simulink library "roller485lib"  (R2023a)
settings: Solver=VariableStepAuto  StartTime=0.0  StopTime=10.0  RelTol=1e-3
libraries: arduinolib x135, simulink x46
(part 4 of 4)

== matlab function roller485lib/I2C Write (using MATLAB Function)/current command [mA] (using MATLAB Function)/MATLAB Function ==
  data: double_data input; bytes output
function bytes = double_to_bytes_uint8(double_data)

bytes        = zeros(1, 4, 'uint8');             % 明示的に型とサイズを宣言
signed_int   = int32(double_data);
unsigned_int = typecast(signed_int, 'uint32');
bytes(1:4)   = typecast(unsigned_int, 'uint8');  % サイズを明示

== matlab function roller485lib/I2C Write (using MATLAB Function)/relative angle command [deg] (using MATLAB Function)/Enabled Subsystem (initialization angle)/MATLAB Function ==
  data: bytes input; double_data output
function double_data = bytes_uint8_to_double(bytes)

double_data    = zeros(1, 1, 'double');    % 明示的に型とサイズを宣言
unsigned_int   = typecast(uint8(bytes), 'uint32');
signed_int     = typecast(unsigned_int, 'int32');
double_data(1) = double(signed_int);       % サイズを明示

== matlab function roller485lib/I2C Write/relative angle command [rad]/Enabled Subsystem (initialization angle)/MATLAB Function ==
  data: bytes input; double_data output
function double_data = bytes_uint8_to_double(bytes)

double_data    = zeros(1, 1, 'double');    % 明示的に型とサイズを宣言
unsigned_int   = typecast(uint8(bytes), 'uint32');
signed_int     = typecast(unsigned_int, 'int32');
double_data(1) = double(signed_int);       % サイズを明示

== matlab function roller485lib/I2C Write (using MATLAB Function)/relative angle command [deg] (using MATLAB Function)/MATLAB Function ==
  data: double_data input; bytes output
function bytes = double_to_bytes_uint8(double_data)

bytes        = zeros(1, 4, 'uint8');             % 明示的に型とサイズを宣言
signed_int   = int32(double_data);
unsigned_int = typecast(signed_int, 'uint32');
bytes(1:4)   = typecast(unsigned_int, 'uint8');  % サイズを明示

== matlab function roller485lib/I2C Write (using MATLAB Function)/relative angle command [rad] (using MATLAB Function)/Enabled Subsystem (initialization angle)/MATLAB Function ==
  data: bytes input; double_data output
function double_data = bytes_uint8_to_double(bytes)

double_data    = zeros(1, 1, 'double');    % 明示的に型とサイズを宣言
unsigned_int   = typecast(uint8(bytes), 'uint32');
signed_int     = typecast(unsigned_int, 'int32');
double_data(1) = double(signed_int);       % サイズを明示

== matlab function roller485lib/I2C Write (using MATLAB Function)/relative angle command [rad] (using MATLAB Function)/MATLAB Function ==
  data: double_data input; bytes output
function bytes = double_to_bytes_uint8(double_data)

bytes        = zeros(1, 4, 'uint8');             % 明示的に型とサイズを宣言
signed_int   = int32(double_data);
unsigned_int = typecast(signed_int, 'uint32');
bytes(1:4)   = typecast(unsigned_int, 'uint8');  % サイズを明示

== matlab function roller485lib/I2C Read (using MATLAB Function)/absolute angle detection [rad] (using MATLAB Function)/MATLAB Function ==
  data: bytes input; double_data output
function double_data = bytes_uint8_to_double(bytes)

double_data    = zeros(1, 1, 'double');    % 明示的に型とサイズを宣言
unsigned_int   = typecast(uint8(bytes), 'uint32');
signed_int     = typecast(unsigned_int, 'int32');
double_data(1) = double(signed_int);       % サイズを明示

== matlab function roller485lib/I2C Read (using MATLAB Function)/relative angle detection [rad] (using MATLAB Function)/MATLAB Function ==
  data: bytes input; double_data output
function double_data = bytes_uint8_to_double(bytes)

double_data    = zeros(1, 1, 'double');    % 明示的に型とサイズを宣言
unsigned_int   = typecast(uint8(bytes), 'uint32');
signed_int     = typecast(unsigned_int, 'int32');
double_data(1) = double(signed_int);       % サイズを明示

== matlab function roller485lib/I2C Read (using MATLAB Function)/absolute angle detection [deg] (using MATLAB Function)/MATLAB Function ==
  data: bytes input; double_data output
function double_data = bytes_uint8_to_double(bytes)

double_data    = zeros(1, 1, 'double');    % 明示的に型とサイズを宣言
unsigned_int   = typecast(uint8(bytes), 'uint32');
signed_int     = typecast(unsigned_int, 'int32');
double_data(1) = double(signed_int);       % サイズを明示

== matlab function roller485lib/I2C Write/relative angle command [deg]/Enabled Subsystem (initialization angle)/MATLAB Function ==
  data: bytes input; double_data output
function double_data = bytes_uint8_to_double(bytes)

double_data    = zeros(1, 1, 'double');    % 明示的に型とサイズを宣言
unsigned_int   = typecast(uint8(bytes), 'uint32');
signed_int     = typecast(unsigned_int, 'int32');
double_data(1) = double(signed_int);       % サイズを明示

== matlab function roller485lib/I2C Read (using MATLAB Function)/angular velocity detection using LPF [rpm] (using MATLAB Function)/MATLAB Function2 ==
  data: bytes input; double_data output
function double_data = bytes_uint8_to_double(bytes)

double_data    = zeros(1, 1, 'double');    % 明示的に型とサイズを宣言
unsigned_int   = typecast(uint8(bytes), 'uint32');
signed_int     = typecast(unsigned_int, 'int32');
double_data(1) = double(signed_int);       % サイズを明示

== matlab function roller485lib/I2C Read (using MATLAB Function)/current detection [mA] (using MATLAB Function)/MATLAB Function ==
  data: bytes input; double_data output
function double_data = bytes_uint8_to_double(bytes)

double_data    = zeros(1, 1, 'double');    % 明示的に型とサイズを宣言
unsigned_int   = typecast(uint8(bytes), 'uint32');
signed_int     = typecast(unsigned_int, 'int32');
double_data(1) = double(signed_int);       % サイズを明示

== matlab function roller485lib/I2C Read (using MATLAB Function)/relative angle detection [deg] (using MATLAB Function)/MATLAB Function ==
  data: bytes input; double_data output
function double_data = bytes_uint8_to_double(bytes)

double_data    = zeros(1, 1, 'double');    % 明示的に型とサイズを宣言
unsigned_int   = typecast(uint8(bytes), 'uint32');
signed_int     = typecast(unsigned_int, 'int32');
double_data(1) = double(signed_int);       % サイズを明示

== matlab function roller485lib/Basic I2C Write (using MATLAB Function)/basic relative angle command [rad] (using MATLAB Function)/Enabled Subsystem (initialization angle)/MATLAB Function ==
  data: bytes input; double_data output
function double_data = bytes_uint8_to_double(bytes)

double_data    = zeros(1, 1, 'double');    % 明示的に型とサイズを宣言
unsigned_int   = typecast(uint8(bytes), 'uint32');
signed_int     = typecast(unsigned_int, 'int32');
double_data(1) = double(signed_int);       % サイズを明示

== matlab function roller485lib/Basic I2C Write (using MATLAB Function)/basic relative angle command [rad] (using MATLAB Function)/MATLAB Function ==
  data: double_data input; bytes output
function bytes = double_to_bytes_uint8(double_data)

bytes        = zeros(1, 4, 'uint8');             % 明示的に型とサイズを宣言
signed_int   = int32(double_data);
unsigned_int = typecast(signed_int, 'uint32');
bytes(1:4)   = typecast(unsigned_int, 'uint8');  % サイズを明示

== matlab function roller485lib/Basic I2C Write (using MATLAB Function)/position PID (using MATLAB Function)/MATLAB Function (D) ==
  data: double_data input; bytes output
function bytes = double_to_bytes_uint8(double_data)

bytes        = zeros(1, 4, 'uint8');             % 明示的に型とサイズを宣言
signed_int   = int32(double_data);
unsigned_int = typecast(signed_int, 'uint32');
bytes(1:4)   = typecast(unsigned_int, 'uint8');  % サイズを明示

== matlab function roller485lib/Basic I2C Write (using MATLAB Function)/position PID (using MATLAB Function)/MATLAB Function (I) ==
  data: double_data input; bytes output
function bytes = double_to_bytes_uint8(double_data)

bytes        = zeros(1, 4, 'uint8');             % 明示的に型とサイズを宣言
signed_int   = int32(double_data);
unsigned_int = typecast(signed_int, 'uint32');
bytes(1:4)   = typecast(unsigned_int, 'uint8');  % サイズを明示

== matlab function roller485lib/Basic I2C Write (using MATLAB Function)/position PID (using MATLAB Function)/MATLAB Function (P) ==
  data: double_data input; bytes output
function bytes = double_to_bytes_uint8(double_data)

bytes        = zeros(1, 4, 'uint8');             % 明示的に型とサイズを宣言
signed_int   = int32(double_data);
unsigned_int = typecast(signed_int, 'uint32');
bytes(1:4)   = typecast(unsigned_int, 'uint8');  % サイズを明示

== matlab function roller485lib/Basic I2C Write (using MATLAB Function)/position PID (within set time) (using MATLAB Function)/Enabled Subsystem/MATLAB Function (D) ==
  data: double_data input; bytes output
function bytes = double_to_bytes_uint8(double_data)

bytes        = zeros(1, 4, 'uint8');             % 明示的に型とサイズを宣言
signed_int   = int32(double_data);
unsigned_int = typecast(signed_int, 'uint32');
bytes(1:4)   = typecast(unsigned_int, 'uint8');  % サイズを明示

== matlab function roller485lib/Basic I2C Write (using MATLAB Function)/position PID (within set time) (using MATLAB Function)/Enabled Subsystem/MATLAB Function (I) ==
  data: double_data input; bytes output
function bytes = double_to_bytes_uint8(double_data)

bytes        = zeros(1, 4, 'uint8');             % 明示的に型とサイズを宣言
signed_int   = int32(double_data);
unsigned_int = typecast(signed_int, 'uint32');
bytes(1:4)   = typecast(unsigned_int, 'uint8');  % サイズを明示

== matlab function roller485lib/I2C Read (using MATLAB Function)/angular velocity detection using LPF [rad//s] (using MATLAB Function)/MATLAB Function2 ==
  data: bytes input; double_data output
function double_data = bytes_uint8_to_double(bytes)

double_data    = zeros(1, 1, 'double');    % 明示的に型とサイズを宣言
unsigned_int   = typecast(uint8(bytes), 'uint32');
signed_int     = typecast(unsigned_int, 'int32');
double_data(1) = double(signed_int);       % サイズを明示

== matlab function roller485lib/Basic I2C Write (using MATLAB Function)/position PID (within set time) (using MATLAB Function)/Enabled Subsystem/MATLAB Function (P) ==
  data: double_data input; bytes output
function bytes = double_to_bytes_uint8(double_data)

bytes        = zeros(1, 4, 'uint8');             % 明示的に型とサイズを宣言
signed_int   = int32(double_data);
unsigned_int = typecast(signed_int, 'uint32');
bytes(1:4)   = typecast(unsigned_int, 'uint8');  % サイズを明示

== matlab function roller485lib/Basic I2C Write (using MATLAB Function)/speed PID (using MATLAB Function)/MATLAB Function (D) ==
  data: double_data input; bytes output
function bytes = double_to_bytes_uint8(double_data)

bytes        = zeros(1, 4, 'uint8');             % 明示的に型とサイズを宣言
signed_int   = int32(double_data);
unsigned_int = typecast(signed_int, 'uint32');
bytes(1:4)   = typecast(unsigned_int, 'uint8');  % サイズを明示

== matlab function roller485lib/Basic I2C Write (using MATLAB Function)/speed PID (using MATLAB Function)/MATLAB Function (I) ==
  data: double_data input; bytes output
function bytes = double_to_bytes_uint8(double_data)

bytes        = zeros(1, 4, 'uint8');             % 明示的に型とサイズを宣言
signed_int   = int32(double_data);
unsigned_int = typecast(signed_int, 'uint32');
bytes(1:4)   = typecast(unsigned_int, 'uint8');  % サイズを明示

== matlab function roller485lib/Basic I2C Write (using MATLAB Function)/speed PID (using MATLAB Function)/MATLAB Function (P) ==
  data: double_data input; bytes output
function bytes = double_to_bytes_uint8(double_data)

bytes        = zeros(1, 4, 'uint8');             % 明示的に型とサイズを宣言
signed_int   = int32(double_data);
unsigned_int = typecast(signed_int, 'uint32');
bytes(1:4)   = typecast(unsigned_int, 'uint8');  % サイズを明示

== matlab function roller485lib/Basic I2C Write (using MATLAB Function)/speed PID (within set time) (using MATLAB Function)/Enabled Subsystem/MATLAB Function (D) ==
  data: double_data input; bytes output
function bytes = double_to_bytes_uint8(double_data)

bytes        = zeros(1, 4, 'uint8');             % 明示的に型とサイズを宣言
signed_int   = int32(double_data);
unsigned_int = typecast(signed_int, 'uint32');
bytes(1:4)   = typecast(unsigned_int, 'uint8');  % サイズを明示

== matlab function roller485lib/Basic I2C Write (using MATLAB Function)/speed PID (within set time) (using MATLAB Function)/Enabled Subsystem/MATLAB Function (I) ==
  data: double_data input; bytes output
function bytes = double_to_bytes_uint8(double_data)

bytes        = zeros(1, 4, 'uint8');             % 明示的に型とサイズを宣言
signed_int   = int32(double_data);
unsigned_int = typecast(signed_int, 'uint32');
bytes(1:4)   = typecast(unsigned_int, 'uint8');  % サイズを明示

== matlab function roller485lib/Basic I2C Write (using MATLAB Function)/speed PID (within set time) (using MATLAB Function)/Enabled Subsystem/MATLAB Function (P) ==
  data: double_data input; bytes output
function bytes = double_to_bytes_uint8(double_data)

bytes        = zeros(1, 4, 'uint8');             % 明示的に型とサイズを宣言
signed_int   = int32(double_data);
unsigned_int = typecast(signed_int, 'uint32');
bytes(1:4)   = typecast(unsigned_int, 'uint8');  % サイズを明示

== matlab function roller485lib/I2C Write (using MATLAB Function)/angular velocity command [rpm] (using MATLAB Function)/Enabled Subsystem (PID setting)/MATLAB Function (P) ==
  data: double_data input; bytes output
function bytes = double_to_bytes_uint8(double_data)

bytes        = zeros(1, 4, 'uint8');             % 明示的に型とサイズを宣言
signed_int   = int32(double_data);
unsigned_int = typecast(signed_int, 'uint32');
bytes(1:4)   = typecast(unsigned_int, 'uint8');  % サイズを明示

== matlab function roller485lib/I2C Write (using MATLAB Function)/angular velocity command [rad//s] (using MATLAB Function)/Enabled Subsystem (PID setting)/MATLAB Function (D) ==
  data: double_data input; bytes output
function bytes = double_to_bytes_uint8(double_data)

bytes        = zeros(1, 4, 'uint8');             % 明示的に型とサイズを宣言
signed_int   = int32(double_data);
unsigned_int = typecast(signed_int, 'uint32');
bytes(1:4)   = typecast(unsigned_int, 'uint8');  % サイズを明示

== matlab function roller485lib/I2C Write (using MATLAB Function)/angular velocity command [rad//s] (using MATLAB Function)/Enabled Subsystem (PID setting)/MATLAB Function (I) ==
  data: double_data input; bytes output
function bytes = double_to_bytes_uint8(double_data)

bytes        = zeros(1, 4, 'uint8');             % 明示的に型とサイズを宣言
signed_int   = int32(double_data);
unsigned_int = typecast(signed_int, 'uint32');
bytes(1:4)   = typecast(unsigned_int, 'uint8');  % サイズを明示

== matlab function roller485lib/I2C Read (using MATLAB Function)/current detection [A] (using MATLAB Function)/MATLAB Function ==
  data: bytes input; double_data output
function double_data = bytes_uint8_to_double(bytes)

double_data    = zeros(1, 1, 'double');    % 明示的に型とサイズを宣言
unsigned_int   = typecast(uint8(bytes), 'uint32');
signed_int     = typecast(unsigned_int, 'int32');
double_data(1) = double(signed_int);       % サイズを明示

== matlab function roller485lib/I2C Write (using MATLAB Function)/angular velocity command [rad//s] (using MATLAB Function)/Enabled Subsystem (PID setting)/MATLAB Function (P) ==
  data: double_data input; bytes output
function bytes = double_to_bytes_uint8(double_data)

bytes        = zeros(1, 4, 'uint8');             % 明示的に型とサイズを宣言
signed_int   = int32(double_data);
unsigned_int = typecast(signed_int, 'uint32');
bytes(1:4)   = typecast(unsigned_int, 'uint8');  % サイズを明示

== matlab function roller485lib/I2C Write (using MATLAB Function)/absolute angle command [deg] (using MATLAB Function)/Enabled Subsystem (PID setting)/MATLAB Function (D) ==
  data: double_data input; bytes output
function bytes = double_to_bytes_uint8(double_data)

bytes        = zeros(1, 4, 'uint8');             % 明示的に型とサイズを宣言
signed_int   = int32(double_data);
unsigned_int = typecast(signed_int, 'uint32');
bytes(1:4)   = typecast(unsigned_int, 'uint8');  % サイズを明示

== matlab function roller485lib/I2C Write (using MATLAB Function)/absolute angle command [deg] (using MATLAB Function)/Enabled Subsystem (PID setting)/MATLAB Function (I) ==
  data: double_data input; bytes output
function bytes = double_to_bytes_uint8(double_data)

bytes        = zeros(1, 4, 'uint8');             % 明示的に型とサイズを宣言
signed_int   = int32(double_data);
unsigned_int = typecast(signed_int, 'uint32');
bytes(1:4)   = typecast(unsigned_int, 'uint8');  % サイズを明示

== matlab function roller485lib/I2C Write (using MATLAB Function)/absolute angle command [deg] (using MATLAB Function)/Enabled Subsystem (PID setting)/MATLAB Function (P) ==
  data: double_data input; bytes output
function bytes = double_to_bytes_uint8(double_data)

bytes        = zeros(1, 4, 'uint8');             % 明示的に型とサイズを宣言
signed_int   = int32(double_data);
unsigned_int = typecast(signed_int, 'uint32');
bytes(1:4)   = typecast(unsigned_int, 'uint8');  % サイズを明示

== matlab function roller485lib/I2C Write (using MATLAB Function)/absolute angle command [rad] (using MATLAB Function)/Enabled Subsystem (PID setting)/MATLAB Function (D) ==
  data: double_data input; bytes output
function bytes = double_to_bytes_uint8(double_data)

bytes        = zeros(1, 4, 'uint8');             % 明示的に型とサイズを宣言
signed_int   = int32(double_data);
unsigned_int = typecast(signed_int, 'uint32');
bytes(1:4)   = typecast(unsigned_int, 'uint8');  % サイズを明示

== matlab function roller485lib/I2C Write (using MATLAB Function)/absolute angle command [rad] (using MATLAB Function)/Enabled Subsystem (PID setting)/MATLAB Function (I) ==
  data: double_data input; bytes output
function bytes = double_to_bytes_uint8(double_data)

bytes        = zeros(1, 4, 'uint8');             % 明示的に型とサイズを宣言
signed_int   = int32(double_data);
unsigned_int = typecast(signed_int, 'uint32');
bytes(1:4)   = typecast(unsigned_int, 'uint8');  % サイズを明示

== matlab function roller485lib/I2C Write (using MATLAB Function)/absolute angle command [rad] (using MATLAB Function)/Enabled Subsystem (PID setting)/MATLAB Function (P) ==
  data: double_data input; bytes output
function bytes = double_to_bytes_uint8(double_data)

bytes        = zeros(1, 4, 'uint8');             % 明示的に型とサイズを宣言
signed_int   = int32(double_data);
unsigned_int = typecast(signed_int, 'uint32');
bytes(1:4)   = typecast(unsigned_int, 'uint8');  % サイズを明示

== matlab function roller485lib/I2C Write (using MATLAB Function)/relative angle command [deg] (using MATLAB Function)/Enabled Subsystem (PID setting)/MATLAB Function (D) ==
  data: double_data input; bytes output
function bytes = double_to_bytes_uint8(double_data)

bytes        = zeros(1, 4, 'uint8');             % 明示的に型とサイズを宣言
signed_int   = int32(double_data);
unsigned_int = typecast(signed_int, 'uint32');
bytes(1:4)   = typecast(unsigned_int, 'uint8');  % サイズを明示

== matlab function roller485lib/I2C Write (using MATLAB Function)/relative angle command [deg] (using MATLAB Function)/Enabled Subsystem (PID setting)/MATLAB Function (I) ==
  data: double_data input; bytes output
function bytes = double_to_bytes_uint8(double_data)

bytes        = zeros(1, 4, 'uint8');             % 明示的に型とサイズを宣言
signed_int   = int32(double_data);
unsigned_int = typecast(signed_int, 'uint32');
bytes(1:4)   = typecast(unsigned_int, 'uint8');  % サイズを明示

== matlab function roller485lib/I2C Write (using MATLAB Function)/relative angle command [deg] (using MATLAB Function)/Enabled Subsystem (PID setting)/MATLAB Function (P) ==
  data: double_data input; bytes output
function bytes = double_to_bytes_uint8(double_data)

bytes        = zeros(1, 4, 'uint8');             % 明示的に型とサイズを宣言
signed_int   = int32(double_data);
unsigned_int = typecast(signed_int, 'uint32');
bytes(1:4)   = typecast(unsigned_int, 'uint8');  % サイズを明示

== matlab function roller485lib/Basic I2C Write (using MATLAB Function)/basic absolute angle command [deg] (using MATLAB Function)/MATLAB Function ==
  data: double_data input; bytes output
function bytes = double_to_bytes_uint8(double_data)

bytes        = zeros(1, 4, 'uint8');             % 明示的に型とサイズを宣言
signed_int   = int32(double_data);
unsigned_int = typecast(signed_int, 'uint32');
bytes(1:4)   = typecast(unsigned_int, 'uint8');  % サイズを明示

== matlab function roller485lib/I2C Write (using MATLAB Function)/relative angle command [rad] (using MATLAB Function)/Enabled Subsystem (PID setting)/MATLAB Function (D) ==
  data: double_data input; bytes output
function bytes = double_to_bytes_uint8(double_data)

bytes        = zeros(1, 4, 'uint8');             % 明示的に型とサイズを宣言
signed_int   = int32(double_data);
unsigned_int = typecast(signed_int, 'uint32');
bytes(1:4)   = typecast(unsigned_int, 'uint8');  % サイズを明示

== matlab function roller485lib/I2C Write (using MATLAB Function)/relative angle command [rad] (using MATLAB Function)/Enabled Subsystem (PID setting)/MATLAB Function (I) ==
  data: double_data input; bytes output
function bytes = double_to_bytes_uint8(double_data)

bytes        = zeros(1, 4, 'uint8');             % 明示的に型とサイズを宣言
signed_int   = int32(double_data);
unsigned_int = typecast(signed_int, 'uint32');
bytes(1:4)   = typecast(unsigned_int, 'uint8');  % サイズを明示

== matlab function roller485lib/I2C Write (using MATLAB Function)/relative angle command [rad] (using MATLAB Function)/Enabled Subsystem (PID setting)/MATLAB Function (P) ==
  data: double_data input; bytes output
function bytes = double_to_bytes_uint8(double_data)

bytes        = zeros(1, 4, 'uint8');             % 明示的に型とサイズを宣言
signed_int   = int32(double_data);
unsigned_int = typecast(signed_int, 'uint32');
bytes(1:4)   = typecast(unsigned_int, 'uint8');  % サイズを明示

== matlab function roller485lib/Basic I2C Write/basic relative angle command [deg]/Enabled Subsystem (initialization angle)/MATLAB Function ==
  data: bytes input; double_data output
function double_data = bytes_uint8_to_double(bytes)

double_data    = zeros(1, 1, 'double');    % 明示的に型とサイズを宣言
unsigned_int   = typecast(uint8(bytes), 'uint32');
signed_int     = typecast(unsigned_int, 'int32');
double_data(1) = double(signed_int);       % サイズを明示

== matlab function roller485lib/Basic I2C Write/basic relative angle command [rad]/Enabled Subsystem (initialization angle)/MATLAB Function ==
  data: bytes input; double_data output
function double_data = bytes_uint8_to_double(bytes)

double_data    = zeros(1, 1, 'double');    % 明示的に型とサイズを宣言
unsigned_int   = typecast(uint8(bytes), 'uint32');
signed_int     = typecast(unsigned_int, 'int32');
double_data(1) = double(signed_int);       % サイズを明示

== matlab function roller485lib/Basic I2C Write (using MATLAB Function)/basic absolute angle command [rad] (using MATLAB Function)/MATLAB Function ==
  data: double_data input; bytes output
function bytes = double_to_bytes_uint8(double_data)

bytes        = zeros(1, 4, 'uint8');             % 明示的に型とサイズを宣言
signed_int   = int32(double_data);
unsigned_int = typecast(signed_int, 'uint32');
bytes(1:4)   = typecast(unsigned_int, 'uint8');  % サイズを明示

== matlab function roller485lib/I2C Write (using MATLAB Function)/angular velocity command [rpm] (using MATLAB Function)/Enabled Subsystem (PID setting)/MATLAB Function (D) ==
  data: double_data input; bytes output
function bytes = double_to_bytes_uint8(double_data)

bytes        = zeros(1, 4, 'uint8');             % 明示的に型とサイズを宣言
signed_int   = int32(double_data);
unsigned_int = typecast(signed_int, 'uint32');
bytes(1:4)   = typecast(unsigned_int, 'uint8');  % サイズを明示

== matlab function roller485lib/I2C Write (using MATLAB Function)/angular velocity command [rpm] (using MATLAB Function)/Enabled Subsystem (PID setting)/MATLAB Function (I) ==
  data: double_data input; bytes output
function bytes = double_to_bytes_uint8(double_data)

bytes        = zeros(1, 4, 'uint8');             % 明示的に型とサイズを宣言
signed_int   = int32(double_data);
unsigned_int = typecast(signed_int, 'uint32');
bytes(1:4)   = typecast(unsigned_int, 'uint8');  % サイズを明示

== matlab function roller485lib/Basic I2C Write (using MATLAB Function)/basic angular velocity command [rad//s] (using MATLAB Function)/MATLAB Function ==
  data: double_data input; bytes output
function bytes = double_to_bytes_uint8(double_data)

bytes        = zeros(1, 4, 'uint8');             % 明示的に型とサイズを宣言
signed_int   = int32(double_data);
unsigned_int = typecast(signed_int, 'uint32');
bytes(1:4)   = typecast(unsigned_int, 'uint8');  % サイズを明示

== matlab function roller485lib/Basic I2C Write (using MATLAB Function)/basic angular velocity command [rpm] (using MATLAB Function)/MATLAB Function ==
  data: double_data input; bytes output
function bytes = double_to_bytes_uint8(double_data)

bytes        = zeros(1, 4, 'uint8');             % 明示的に型とサイズを宣言
signed_int   = int32(double_data);
unsigned_int = typecast(signed_int, 'uint32');
bytes(1:4)   = typecast(unsigned_int, 'uint8');  % サイズを明示

== matlab function roller485lib/Basic I2C Write (using MATLAB Function)/basic current command [A] (using MATLAB Function)/MATLAB Function ==
  data: double_data input; bytes output
function bytes = double_to_bytes_uint8(double_data)

bytes        = zeros(1, 4, 'uint8');             % 明示的に型とサイズを宣言
signed_int   = int32(double_data);
unsigned_int = typecast(signed_int, 'uint32');
bytes(1:4)   = typecast(unsigned_int, 'uint8');  % サイズを明示

== matlab function roller485lib/Basic I2C Write (using MATLAB Function)/basic current command [mA] (using MATLAB Function)/MATLAB Function ==
  data: double_data input; bytes output
function bytes = double_to_bytes_uint8(double_data)

bytes        = zeros(1, 4, 'uint8');             % 明示的に型とサイズを宣言
signed_int   = int32(double_data);
unsigned_int = typecast(signed_int, 'uint32');
bytes(1:4)   = typecast(unsigned_int, 'uint8');  % サイズを明示

== matlab function roller485lib/Basic I2C Write (using MATLAB Function)/basic relative angle command [deg] (using MATLAB Function)/Enabled Subsystem (initialization angle)/MATLAB Function ==
  data: bytes input; double_data output
function double_data = bytes_uint8_to_double(bytes)

double_data    = zeros(1, 1, 'double');    % 明示的に型とサイズを宣言
unsigned_int   = typecast(uint8(bytes), 'uint32');
signed_int     = typecast(unsigned_int, 'int32');
double_data(1) = double(signed_int);       % サイズを明示
